simulink model "simulink_computer_auto_highlighted"  (R2022b)
settings: Solver=VariableStepAuto  StartTime=0.0  StopTime=inf  RelTol=1e-3
libraries: simulink_extras x21, dspswit3 x1, simulink x1, hdlsllib x1
(part 1 of 2)
settings Model: Creator=F1  LastModifiedBy=Namratha
settings SolverCC: AlgebraicLoopSolver=TrustRegion
settings OptimizationCC: BooleanDataType=off
settings DebuggingCC: UnconnectedInputMsg=warning  UnconnectedOutputMsg=warning  UnconnectedLineMsg=warning  SFMachineParentedDataDiag=warning
settings ModelReferenceCC: EnableRefExpFcnMdlSchedulingChecks=on

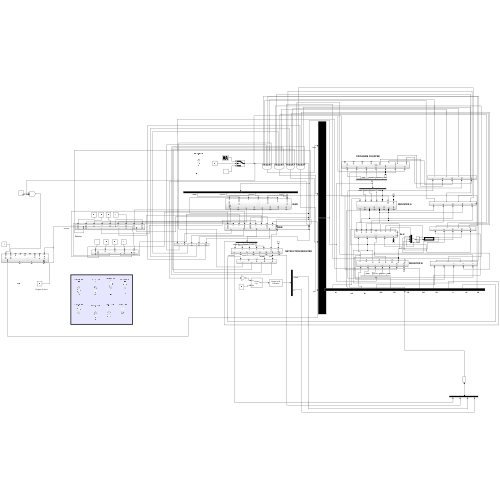
[thumbnail: Simulink's stored preview of the top-level diagram]
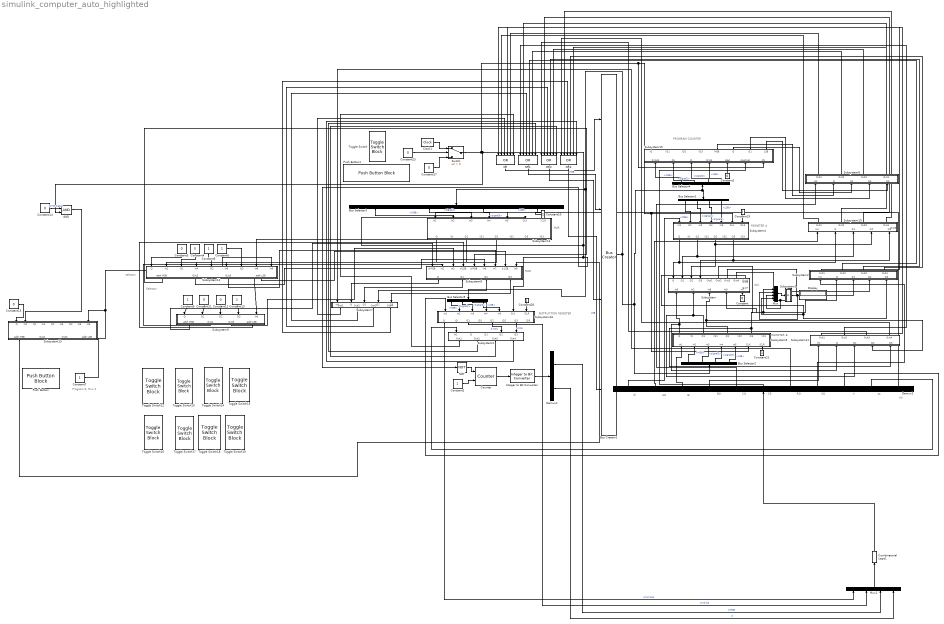
== system simulink_computer_auto_highlighted ==
  note: selector
  note: MI
  note: IO
  note: II
  note: SO
  note: RO
  note: CE
  note: CO
  note: BO
  note: BI
  note: AO
  note: AI
  note: MAR
  note: Program:0, Run:1
  note: ALU
  note: REGISTER B
  note: REGISTER A
  note: PROGRAM COUNTER
  note: RAM
  note: Selector
  note: INSTRUCTION REGISTER
  AND : Logic  IconShape=distinctive  AllPortsSameDT=off  OutDataTypeStr=boolean
  Bus Creator1 : BusCreator  Inputs=4
  Bus Selector{1..5} (5 alike) : BusSelector  OutputSignals=MSB,signal2,signal3,LSB
  Clock1 : simulink_extras/Flip Flops/Clock  period=2
  Combinatorial Logic1 : CombinatorialLogic  TruthTable=|
      | [0	0	0	0	1	0	0	0	0	0	1;
      | 0	0	0	0	0	1	1	0	1	0	0;
      | 0	0	0	0	0	0	0	0	0	1	1;
      | 1	0	0	0	0	0	1	0	0	0	0;
      | 0	0	0	0	1	0	0	0	0	0	1;
      | 0	0	0	0	0	1	1	0	1	0	0;
      | 0	0	1	0	0	0	0	0	0	1	0;
      | 0	0	0	0	0	0	0	0	0	0	0;
      | 0	0	0	0	1	0	0	0	0	0	1;
      | 0	0	0	0	0	1	1	0	1	0	0;
      | 0	0	1	0	0	0	0	1	0	0	0;
      | 0	0	0	0	0	0	0	0	0	0	0;
      | 0	0	0	0	0	0	0	0	0	0	0;
      | 0	0	0	0	0	0	0	0	0	0	0;
      | 0	0	0	0	0	0	0	0	0	0	0;
      | 0	0	0	0	0	0	0	0	0	0	0]
  Constant{,1,14..15,17,23} (6 alike) : Constant  Value=0
  Constant{2,10,19,21,28} (5 alike) : Constant
  Constant{3..4,11..12} (4 alike) : Constant  Value=0  OutDataTypeStr=boolean  LockScale=on
  Constant{5..7,9,13} (5 alike) : Constant  OutDataTypeStr=boolean  LockScale=on
  Counter : dspswit3/Counter  Direction=Up  CountEvent=Rising edge  CounterSize=User defined  MaxCount=3  InitialCount=0  Output=Count  HitValue=32  ResetInput=on  SamplesPerFrame=1  Ts=1  CntDtype=int16  HitDtype=Logical
  Demux1 : Demux  Outputs=2
  Demux2 : Demux  Outputs=11
  Display : Display
  Integer to Bit Converter : simulink/Logic and Bit Operations/Integer to Bit Converter  nbits=2  signedInputValues=Unsigned  bitOrder=MSB first  outDtype=boolean
      settings: LibrarySourceBlock=|
      | commutil2/Integer to Bit
      | Converter
  Mux : Mux
  Mux1 : Mux
  NOT : Logic  Operator=NOT  IconShape=distinctive  AllPortsSameDT=off  OutDataTypeStr=boolean
  OR{,1..3} (4 alike) : Logic  Operator=OR  Inputs=6  IconShape=distinctive  AllPortsSameDT=off  OutDataTypeStr=boolean
  Push Button : PushButtonBlock  OffValue=0.000000
  Push Button1 : PushButtonBlock  OffValue=0.000000
  Subsystem : Subsystem
      settings: PortSchema="{\"entries\":[{\"content\":{\"sides\":[{\"content\":{\"connectorIds\":[\"In1\",\"In2\",\"In3\",\"In4\",\"In5\"]},\"type\":\"ConnectorPlacement.EquallySpacedRectSide\",\"uuid\":\"d76b9681-1e35-4330-834d-a6fb8ece3ca6\"},{\"content\":{\"connectorIds\":[\"In6\",\"In7\",\"In8\",\"In9\",\"Out1\",\"Out2\",\"Out3\",\"Out4\",\"Out5\"],\"side\":\"RIGHT\"},\"type\":\"ConnectorPlacement.EquallySpacedRectSide\",\"uuid\":\"5f7e2d0d-b340-42cb-b0df-c47f3adaa3c8\"},{\"content\":{\"connectorIds\":[],\"side\":\"TOP\"},\"type\":\"ConnectorPlacement.EquallySpacedRectSide\",\"uuid\":\"9ba6019d-435d-4d43-af51-5a6472d9473c\"},{\"content\":{\"connectorIds\":[\"Out6\",\"Out7\"],\"side\":\"BOTTOM\"},\"type\":\"ConnectorPlacement.EquallySpacedRectSide\",\"uuid\":\"ff52050d-6b1c-4dc9-b693-b127a6983cae\"}]},\"type\":\"ConnectorPlacement.EquallySpacedConnector\",\"uuid\":\"63f40923-5384-474a-9ba8-b1a2be7f0fa2\"}],\"packageUris\":[\"http://schema.mathworks.com/mf0/Connector/R2020b\"],\"version\":\"1.0\"}"
  Subsystem1 : Subsystem
  Subsystem10 : Subsystem
      settings: PortSchema="{\"entries\":[{\"content\":{\"sides\":[{\"content\":{\"connectorIds\":[\"In1\",\"In2\",\"In3\",\"In4\",\"In5\"]},\"type\":\"ConnectorPlacement.EquallySpacedRectSide\",\"uuid\":\"be1d6c7a-a71e-4dd8-8c15-a91081576af0\"},{\"content\":{\"connectorIds\":[\"Out1\",\"Out2\",\"Out3\",\"Out4\"],\"side\":\"RIGHT\"},\"type\":\"ConnectorPlacement.EquallySpacedRectSide\",\"uuid\":\"047de8eb-1583-4af5-9052-d7fc7813080f\"},{\"content\":{\"connectorIds\":[],\"side\":\"TOP\"},\"type\":\"ConnectorPlacement.EquallySpacedRectSide\",\"uuid\":\"384f979b-6520-4a26-a075-1614f2aab292\"},{\"content\":{\"connectorIds\":[\"Out5\"],\"side\":\"BOTTOM\"},\"type\":\"ConnectorPlacement.EquallySpacedRectSide\",\"uuid\":\"fda4a962-651a-4873-b6d0-34c5738e96d2\"}]},\"type\":\"ConnectorPlacement.EquallySpacedConnector\",\"uuid\":\"d67f7e62-ac02-4d91-8456-d744cd866721\"}],\"packageUris\":[\"http://schema.mathworks.com/mf0/Connector/R2020b\"],\"version\":\"1.0\"}"
  Subsystem11 : Subsystem
  Subsystem12 : Subsystem
  Subsystem13 : Subsystem
  Subsystem14 : Subsystem
  Subsystem15 : Subsystem
  Subsystem16 : Subsystem
  Subsystem2 : Subsystem
  Subsystem3 : Subsystem
  Subsystem4 : Subsystem
  Subsystem5 : Subsystem
  Subsystem6 : Subsystem
  Subsystem7 : Subsystem
  Subsystem8 : Subsystem
  Subsystem9 : Subsystem
  Switch : Switch  Criteria=u2 > Threshold  SaturateOnIntegerOverflow=off  InputSameDT=off
  Toggle Switch{,12..19} (9 alike) : ToggleSwitchBlock
      settings: Values={{'Off', 'On'}, [0 1]}
  wires:
  Subsystem11/3(Out3) -> OR2/1
  Subsystem7/4(Out4) -> OR3/3
  Subsystem10/1(Out1) -> OR/2
  Subsystem11/4(Out4) -> OR3/1
  Subsystem4/3(Q1) -> Subsystem/7(Q1), Subsystem10/3(Q1)
  Bus Selector1/1 -> Subsystem4/2(In2)  "<MSB>"
  OR/1 -> Bus Creator1/1  "MSB"
  Subsystem7/1(Out1) -> OR/3
  Constant21/1 -> Subsystem5/7(!CLR)
  OR3/1 -> Bus Creator1/4  "LSB"
  Constant19/1 -> Subsystem4/7(!CLR)
  Bus Selector2/2 -> Subsystem5/3(In3)  "<signal2>"
  Bus Selector2/4 -> Subsystem5/5(In5)  "<LSB>"
  Bus Selector1/2 -> Subsystem4/3(In3)  "<signal2>"
  OR1/1 -> Bus Creator1/2
  Bus Selector1/3 -> Subsystem4/4(In4)  "<signal3>"
  Subsystem4/1(Q) -> Subsystem/6(Q), Subsystem10/2(Q)
  Subsystem7/2(Out2) -> OR1/3
  Subsystem7/3(Out3) -> OR2/3
  Subsystem10/4(Out4) -> OR3/2
  Subsystem4/7(Q3) -> Subsystem/9(Q3), Subsystem10/5(Q3)
  Subsystem5/7(Q3) -> Subsystem/4(In9), Subsystem11/5(Q3)
  Subsystem10/3(Out3) -> OR2/2
  Subsystem4/5(Q2) -> Subsystem/8(Q2), Subsystem10/4(Q2)
  Subsystem10/2(Out2) -> OR1/2
  Subsystem11/1(Out1) -> OR/1
  Subsystem5/5(Q2) -> Subsystem/3(In8), Subsystem11/4(Q2)
  Bus Selector2/1 -> Subsystem5/2(In2)  "<MSB>"
  Bus Selector1/4 -> Subsystem4/5(In5)  "<LSB>"
  Bus Selector2/3 -> Subsystem5/4(In4)  "<signal3>"
  Subsystem5/1(Q) -> Subsystem/1(In6), Subsystem11/2(Q)
  Subsystem5/3(Q1) -> Subsystem11/3(Q1), Subsystem/2(In2)
  OR2/1 -> Bus Creator1/3
  Subsystem11/2(Out2) -> OR1/1
  Constant/1 -> Subsystem/5(In7)
  Subsystem/2(Out2) -> Subsystem2/2(Q), Mux/1
  Subsystem/3(Out3) -> Mux/2, Subsystem2/3(Q1)
  Subsystem/4(Out4) -> Subsystem2/4(Q2), Mux/3
  Subsystem/5(Out5) -> Subsystem2/5(Q3), Mux/4
  Mux/1 -> Subsystem1/1(In1)
  Subsystem1/1(y) -> Display/1
  Demux2/8 -> Subsystem2/1(In1)
  Subsystem2/1(Out1) -> OR/4
  Subsystem2/2(Out2) -> OR1/4
  Subsystem2/3(Out3) -> OR2/4
  Subsystem2/4(Out4) -> OR3/4
  Subsystem6/4(Out4) -> OR3/5
  Subsystem6/3(Out3) -> OR2/5
  Subsystem6/2(Out2) -> OR1/5
  Subsystem6/1(Out1) -> OR/5
  Subsystem12/2(Out2) -> Subsystem8/6(In6)
  Subsystem12/4(addr LSB) -> Subsystem8/8(a LSB)
  Subsystem12/3(Out3) -> Subsystem8/7(In7)
  Subsystem12/1(addr MSB) -> Subsystem8/5(a MSB)
  Constant3/1 -> Subsystem12/1(Q)
  Constant4/1 -> Subsystem12/3(Q1)
  Constant5/1 -> Subsystem12/5(Q2)
  Constant6/1 -> Subsystem12/7(Q3)
  Bus Selector3/1 -> Subsystem14/2(In2)  "<MSB>"
  Bus Selector3/4 -> Subsystem14/5(In5)  "<LSB>"
  Bus Selector3/2 -> Subsystem14/3(In3)  "<signal2>"
  Bus Selector3/3 -> Subsystem14/4(In4)  "<signal3>"
  Subsystem14/1(Q) -> Subsystem12/2(In2)
  Subsystem14/3(Q1) -> Subsystem12/4(In4)
  Subsystem14/5(Q2) -> Subsystem12/6(In6)
  Subsystem14/7(Q3) -> Subsystem12/8(In8)
  Constant7/1 -> Subsystem13/9(In9), Subsystem9/5(In9), Subsystem12/9(In9)
  Constant10/1 -> Subsystem14/7(!CLR)
  Subsystem9/1(addr MSB) -> Subsystem8/1(d MSB)
  Subsystem9/2(Out2) -> Subsystem8/2(In2)
  Subsystem9/3(Out3) -> Subsystem8/3(In3)
  Subsystem9/4(addr LSB) -> Subsystem8/4(d LSB)
  Constant9/1 -> Subsystem9/1(Q)
  Constant11/1 -> Subsystem9/2(Q1)
  Constant12/1 -> Subsystem9/3(Q2)
  Constant13/1 -> Subsystem9/4(Q3)
  Constant15/1 -> Subsystem13/1(Q)
  Constant14/1 -> AND/1  "Write signal"
  AND/1 -> Subsystem13/2(In2)
  Subsystem13/1(addr MSB) -> Subsystem8/9(In9)
  Constant17/1 -> Switch/3
  Clock1/1 -> Switch/1
  Constant23/1 -> Switch/2
  Subsystem15/5(MSB) -> Subsystem6/2(Q)
  Subsystem15/6(Q) -> Subsystem6/3(Q1)
  Subsystem15/7(Q1) -> Subsystem6/4(Q2)
  Subsystem15/8(LSB) -> Subsystem6/5(Q3)
  Bus Selector4/1 -> Subsystem15/1(D msb)  "<MSB>"
  Bus Selector4/2 -> Subsystem15/2(D1)  "<signal2>"
  Bus Selector4/3 -> Subsystem15/3(D)  "<signal3>"
  Bus Selector4/4 -> Subsystem15/4(D lsb)  "<LSB>"
  Subsystem8/2(Q1) -> Subsystem7/3(Q1)
  Subsystem8/3(Q2) -> Subsystem7/4(Q2)
  Subsystem8/4(Q3) -> Subsystem7/5(Q3)
  Constant28/1 -> Subsystem16/7(!CLR)
  Bus Selector5/3 -> Subsystem16/4(In4)  "<signal3>"
  Bus Selector5/2 -> Subsystem16/3(In3)  "<signal2>"
  Bus Selector5/1 -> Subsystem16/2(In2)  "<MSB>"
  Bus Selector5/4 -> Subsystem16/5(In5)  "<LSB>"
  Subsystem16/5(Q2) -> Subsystem3/4(Q2)  "d msb"
  Subsystem16/7(Q3) -> Subsystem3/5(Q3)  "d lsb"
  Switch/1 -> Subsystem14/6(CLK), Subsystem16/6(CLK), NOT/1, AND/2, Subsystem4/6(CLK), Subsystem5/6(CLK), Subsystem15/7(clk)
  Bus Creator1/1 -> Bus Selector1/1, Bus Selector4/1, Bus Selector2/1, Bus Selector5/1, Bus Selector3/1
  Subsystem3/1(Out1) -> OR/6
  Subsystem3/2(Out2) -> OR1/6
  Subsystem3/3(Out3) -> OR2/6
  Subsystem3/4(Out4) -> OR3/6
  Counter/1 -> Integer to Bit Converter/1
  Integer to Bit Converter/1 -> Demux1/1
  Combinatorial Logic1/1 -> Demux2/1
  Mux1/1 -> Combinatorial Logic1/1
  NOT/1 -> Counter/1
  Constant2/1 -> Counter/2
  Demux1/1 -> Mux1/3  "d MSB"
  Demux1/2 -> Mux1/4  "d"
  Subsystem16/1(Q) -> Mux1/1  "cmd msb"
  Subsystem16/3(Q1) -> Mux1/2  "cmd lsb"
  Demux2/3 -> Subsystem5/1(In1)
  Demux2/1 -> Subsystem4/1(In1)
  Demux2/4 -> Subsystem11/1(In1)
  Demux2/2 -> Subsystem10/1(In1)
  Demux2/6 -> Subsystem15/6(count en)
  Demux2/5 -> Subsystem6/1(In1)
  Demux2/7 -> Subsystem7/1(In1)
  Subsystem8/1(Q) -> Subsystem7/2(Q)
  Demux2/9 -> Subsystem16/1(In1)
  Demux2/11 -> Subsystem14/1(In1)
  Demux2/10 -> Subsystem3/1(In1)
  Constant1/1 -> Subsystem15/5(load)

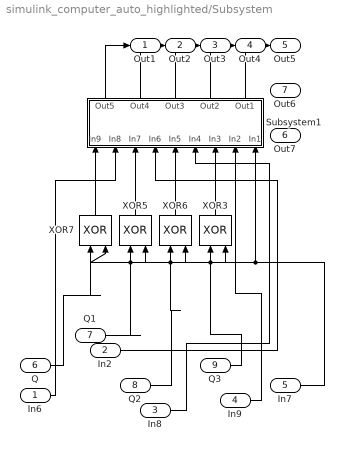
== system simulink_computer_auto_highlighted/Subsystem ==
  In6 : Inport
  In2 : Inport  Port=2
  In8 : Inport  Port=3
  In9 : Inport  Port=4
  In7 : Inport  Port=5
  Q : Inport  Port=6
  Q1 : Inport  Port=7
  Q2 : Inport  Port=8
  Q3 : Inport  Port=9
  Subsystem1 : Subsystem
  XOR{3,5..7} (4 alike) : Logic  Operator=XOR  IconShape=distinctive  AllPortsSameDT=off  OutDataTypeStr=boolean
  Out1 : Outport
  Out2 : Outport  Port=2
  Out3 : Outport  Port=3
  Out4 : Outport  Port=4
  Out5 : Outport  Port=5
  Out7 : Outport  Port=6
  Out6 : Outport  Port=7
  wires:
  XOR6/1 -> Subsystem1/5(In5)
  XOR5/1 -> Subsystem1/7(In7)
  XOR3/1 -> Subsystem1/3(In3)
  Subsystem1/1(Out1) -> Out5/1
  In7/1 -> XOR7/1, XOR5/1, XOR6/1, XOR3/1, Subsystem1/1(In1)
  Subsystem1/2(Out2) -> Out4/1
  Subsystem1/4(Out4) -> Out2/1
  Subsystem1/3(Out3) -> Out3/1
  In2/1 -> Subsystem1/6(In6)
  XOR7/1 -> Subsystem1/9(In9)
  Subsystem1/5(Out5) -> Out1/1
  Q3/1 -> XOR3/2
  Q1/1 -> XOR5/2
  Q/1 -> XOR7/2
  In6/1 -> Subsystem1/8(In8)
  In9/1 -> Subsystem1/2(In2)
  Q2/1 -> XOR6/2
  In8/1 -> Subsystem1/4(In4)

== system simulink_computer_auto_highlighted/Subsystem1 ==
  In1 : Inport
  Demux : Demux
  MATLAB Function : MATLAB Function  TreatAsAtomicUnit=on
  y : Outport
  wires:
  Demux/3 -> MATLAB Function/3(b1)
  Demux/1 -> MATLAB Function/1(b3)
  Demux/2 -> MATLAB Function/2(b2)
  Demux/4 -> MATLAB Function/4(b0)
  MATLAB Function/1(y) -> y/1
  In1/1 -> Demux/1

== system simulink_computer_auto_highlighted/Subsystem10 ==
  In1 : Inport
  Q : Inport  Port=2
  Q1 : Inport  Port=3
  Q2 : Inport  Port=4
  Q3 : Inport  Port=5
  AND{,1..3} (4 alike) : Logic  IconShape=distinctive  AllPortsSameDT=off  OutDataTypeStr=boolean
  Out1 : Outport
  Out2 : Outport  Port=2
  Out3 : Outport  Port=3
  Out4 : Outport  Port=4
  Out5 : Outport  Port=5
  wires:
  In1/1 -> AND3/1, AND2/1, AND1/1, AND/1
  AND1/1 -> Out2/1
  AND3/1 -> Out4/1
  AND/1 -> Out1/1
  Q3/1 -> AND3/2
  Q2/1 -> AND2/2
  Q/1 -> AND/2
  AND2/1 -> Out3/1
  Q1/1 -> AND1/2

== system simulink_computer_auto_highlighted/Subsystem11 ==
  In1 : Inport
  Q : Inport  Port=2
  Q1 : Inport  Port=3
  Q2 : Inport  Port=4
  Q3 : Inport  Port=5
  AND{,1..3} (4 alike) : Logic  IconShape=distinctive  AllPortsSameDT=off  OutDataTypeStr=boolean
  Out1 : Outport
  Out2 : Outport  Port=2
  Out3 : Outport  Port=3
  Out4 : Outport  Port=4
  wires:
  In1/1 -> AND3/1, AND2/1, AND1/1, AND/1
  AND1/1 -> Out2/1
  AND3/1 -> Out4/1
  AND/1 -> Out1/1
  Q3/1 -> AND3/2
  Q2/1 -> AND2/2
  Q/1 -> AND/2
  AND2/1 -> Out3/1
  Q1/1 -> AND1/2

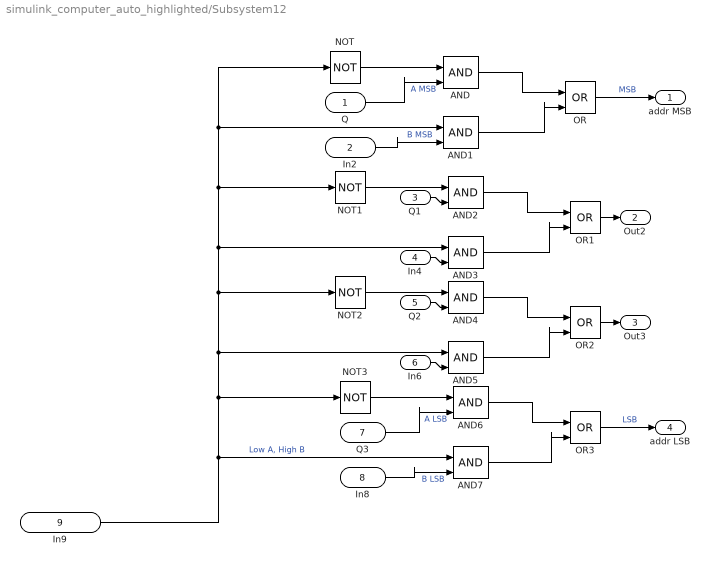
== system simulink_computer_auto_highlighted/Subsystem12 ==
  Q : Inport
  In2 : Inport  Port=2
  Q1 : Inport  Port=3
  In4 : Inport  Port=4
  Q2 : Inport  Port=5
  In6 : Inport  Port=6
  Q3 : Inport  Port=7
  In8 : Inport  Port=8
  In9 : Inport  Port=9
  AND{,1..7} (8 alike) : Logic  IconShape=distinctive  AllPortsSameDT=off  OutDataTypeStr=boolean
  NOT{,1..3} (4 alike) : Logic  Operator=NOT  IconShape=distinctive  AllPortsSameDT=off  OutDataTypeStr=boolean
  OR{,1..3} (4 alike) : Logic  Operator=OR  IconShape=distinctive  AllPortsSameDT=off  OutDataTypeStr=boolean
  addr MSB : Outport
  Out2 : Outport  Port=2
  Out3 : Outport  Port=3
  addr LSB : Outport  Port=4
  wires:
  In9/1 -> AND7/1, NOT3/1, AND5/1, NOT2/1, NOT1/1, AND1/1, NOT/1, AND3/1  "Low A, High B"
  AND5/1 -> OR2/2
  NOT/1 -> AND/1
  NOT1/1 -> AND2/1
  AND/1 -> OR/1
  AND2/1 -> OR1/1
  In4/1 -> AND3/2
  NOT2/1 -> AND4/1
  AND3/1 -> OR1/2
  AND4/1 -> OR2/1
  OR1/1 -> Out2/1
  Q2/1 -> AND4/2
  AND7/1 -> OR3/2
  AND1/1 -> OR/2
  OR/1 -> addr MSB/1  "MSB"
  AND6/1 -> OR3/1
  Q1/1 -> AND2/2
  OR2/1 -> Out3/1
  NOT3/1 -> AND6/1
  In2/1 -> AND1/2  "B MSB"
  In6/1 -> AND5/2
  Q/1 -> AND/2  "A MSB"
  In8/1 -> AND7/2  "B LSB"
  Q3/1 -> AND6/2  "A LSB"
  OR3/1 -> addr LSB/1  "LSB"

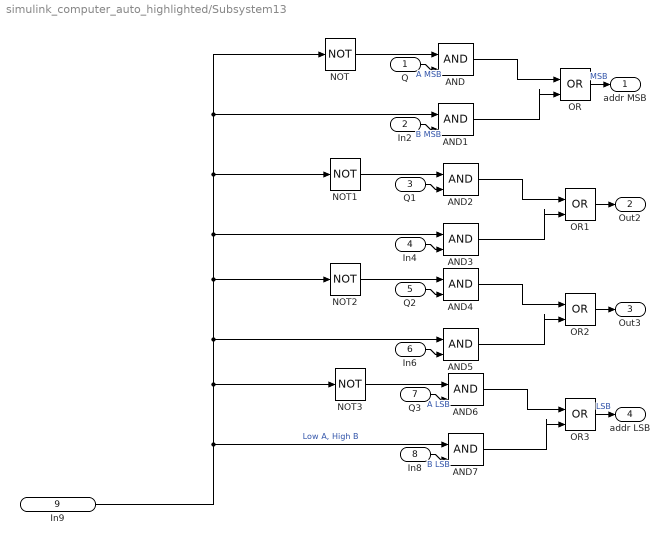
== system simulink_computer_auto_highlighted/Subsystem13 ==
  Q : Inport
  In2 : Inport  Port=2
  Q1 : Inport  Port=3
  In4 : Inport  Port=4
  Q2 : Inport  Port=5
  In6 : Inport  Port=6
  Q3 : Inport  Port=7
  In8 : Inport  Port=8
  In9 : Inport  Port=9
  AND{,1..7} (8 alike) : Logic  IconShape=distinctive  AllPortsSameDT=off  OutDataTypeStr=boolean
  NOT{,1..3} (4 alike) : Logic  Operator=NOT  IconShape=distinctive  AllPortsSameDT=off  OutDataTypeStr=boolean
  OR{,1..3} (4 alike) : Logic  Operator=OR  IconShape=distinctive  AllPortsSameDT=off  OutDataTypeStr=boolean
  addr MSB : Outport
  Out2 : Outport  Port=2
  Out3 : Outport  Port=3
  addr LSB : Outport  Port=4
  wires:
  In9/1 -> AND7/1, NOT3/1, AND5/1, NOT2/1, NOT1/1, AND1/1, NOT/1, AND3/1  "Low A, High B"
  AND5/1 -> OR2/2
  NOT/1 -> AND/1
  NOT1/1 -> AND2/1
  AND/1 -> OR/1
  AND2/1 -> OR1/1
  In4/1 -> AND3/2
  NOT2/1 -> AND4/1
  AND3/1 -> OR1/2
  AND4/1 -> OR2/1
  OR1/1 -> Out2/1
  Q2/1 -> AND4/2
  AND7/1 -> OR3/2
  AND1/1 -> OR/2
  OR/1 -> addr MSB/1  "MSB"
  AND6/1 -> OR3/1
  Q1/1 -> AND2/2
  OR2/1 -> Out3/1
  NOT3/1 -> AND6/1
  In2/1 -> AND1/2  "B MSB"
  In6/1 -> AND5/2
  Q/1 -> AND/2  "A MSB"
  In8/1 -> AND7/2  "B LSB"
  Q3/1 -> AND6/2  "A LSB"
  OR3/1 -> addr LSB/1  "LSB"

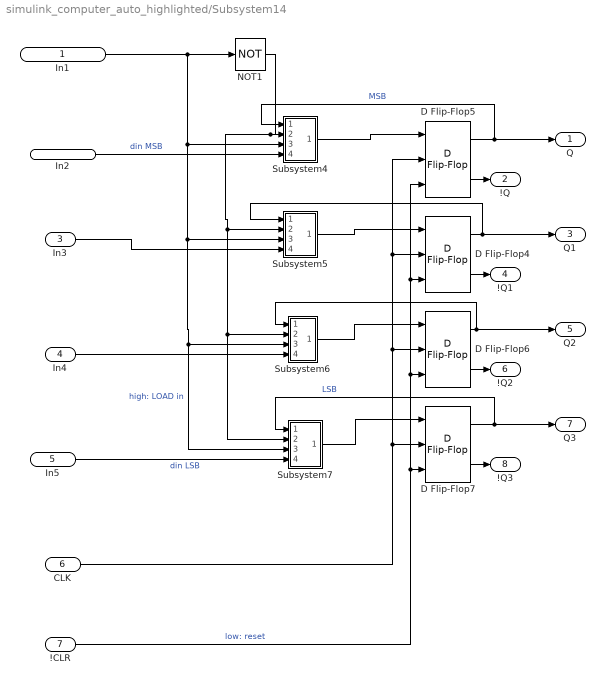
== system simulink_computer_auto_highlighted/Subsystem14 ==
  In1 : Inport
  In2 : Inport  Port=2
  In3 : Inport  Port=3
  In4 : Inport  Port=4
  In5 : Inport  Port=5
  CLK : Inport  Port=6
  !CLR : Inport  Port=7
  D Flip-Flop{4..7} (4 alike) : simulink_extras/Flip Flops/D Flip-Flop
  NOT1 : Logic  Operator=NOT  IconShape=distinctive  AllPortsSameDT=off  OutDataTypeStr=boolean
  Subsystem4 : Subsystem
  Subsystem5 : Subsystem
  Subsystem6 : Subsystem
  Subsystem7 : Subsystem
  Q : Outport
  !Q : Outport  Port=2
  Q1 : Outport  Port=3
  !Q1 : Outport  Port=4
  Q2 : Outport  Port=5
  !Q2 : Outport  Port=6
  Q3 : Outport  Port=7
  !Q3 : Outport  Port=8
  wires:
  In5/1 -> Subsystem7/4(In4)  "din LSB"
  D Flip-Flop5/1 -> Q/1, Subsystem4/1(In1)  "MSB"
  NOT1/1 -> Subsystem7/2(In2), Subsystem6/2(In2), Subsystem5/2(In1), Subsystem4/2(In2)
  Subsystem4/1(Out1) -> D Flip-Flop5/1
  Subsystem7/1(Out1) -> D Flip-Flop7/1
  In3/1 -> Subsystem5/4(In4)
  D Flip-Flop4/2 -> !Q1/1
  D Flip-Flop4/1 -> Q1/1, Subsystem5/1(In2)
  D Flip-Flop7/2 -> !Q3/1
  D Flip-Flop7/1 -> Q3/1, Subsystem7/1(In1)  "LSB"
  D Flip-Flop5/2 -> !Q/1
  Subsystem5/1(Out1) -> D Flip-Flop4/1
  D Flip-Flop6/2 -> !Q2/1
  Subsystem6/1(Out1) -> D Flip-Flop6/1
  D Flip-Flop6/1 -> Q2/1, Subsystem6/1(In1)
  In1/1 -> Subsystem7/3(In3), Subsystem6/3(In3), Subsystem5/3(In3), Subsystem4/3(In3), NOT1/1  "high: LOAD in"
  !CLR/1 -> D Flip-Flop5/3, D Flip-Flop4/3, D Flip-Flop6/3, D Flip-Flop7/3  "low: reset"
  CLK/1 -> D Flip-Flop5/2, D Flip-Flop4/2, D Flip-Flop6/2, D Flip-Flop7/2
  In2/1 -> Subsystem4/4(In4)  "din MSB"
  In4/1 -> Subsystem6/4(In4)

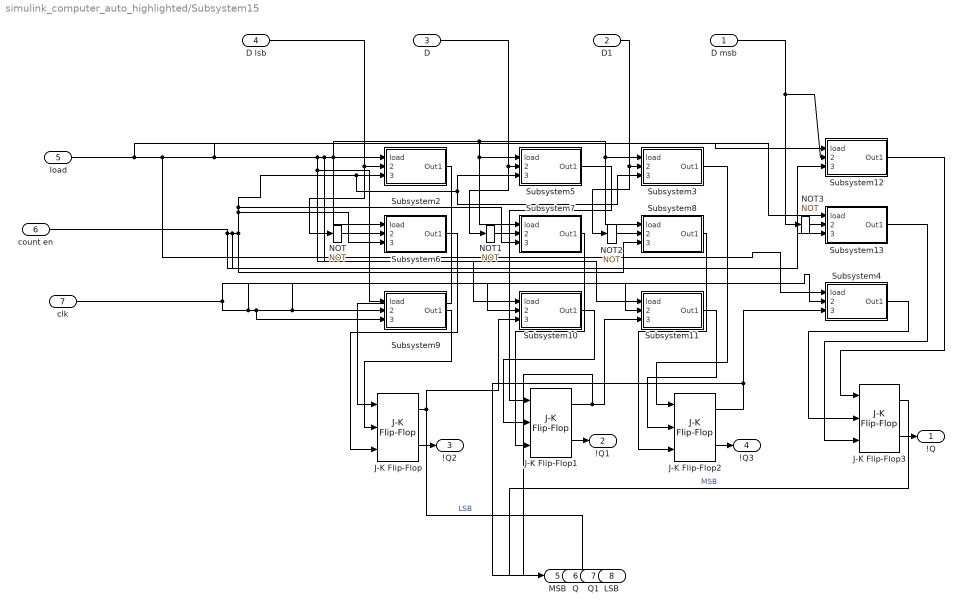
== system simulink_computer_auto_highlighted/Subsystem15 ==
  D msb : Inport
  D1 : Inport  Port=2
  D : Inport  Port=3
  D lsb : Inport  Port=4
  load : Inport  Port=5
  count en : Inport  Port=6
  clk : Inport  Port=7
  J-K Flip-Flop{,1..3} (4 alike) : simulink_extras/Flip Flops/J-K Flip-Flop  initial_condition=0
  NOT{,1..3} (4 alike) : Logic  Operator=NOT  IconShape=distinctive  AllPortsSameDT=off  OutDataTypeStr=boolean
  Subsystem10 : Subsystem
  Subsystem11 : Subsystem
  Subsystem12 : Subsystem
  Subsystem13 : Subsystem
  Subsystem2 : Subsystem
  Subsystem3 : Subsystem
  Subsystem4 : Subsystem
  Subsystem5 : Subsystem
  Subsystem6 : Subsystem
  Subsystem7 : Subsystem
  Subsystem8 : Subsystem
  Subsystem9 : Subsystem
  !Q : Outport
  !Q1 : Outport  Port=2
  !Q2 : Outport  Port=3
  !Q3 : Outport  Port=4
  MSB : Outport  Port=5
  Q : Outport  Port=6
  Q1 : Outport  Port=7
  LSB : Outport  Port=8
  wires:
  count en/1 -> Subsystem12/3(select low), Subsystem13/3(select low), Subsystem5/3(select low), Subsystem3/3(select low), Subsystem2/3(select low), Subsystem7/3(select low), Subsystem6/3(select low), Subsystem8/3(select low)
  clk/1 -> Subsystem11/2(select high), Subsystem9/3(select low), Subsystem4/2(select high), Subsystem9/2(select high), Subsystem10/2(select high)
  Subsystem4/1(Out1) -> J-K Flip-Flop3/2
  Subsystem9/1(Out1) -> J-K Flip-Flop/2
  NOT2/1 -> Subsystem8/2(select high)
  Subsystem13/1(Out1) -> J-K Flip-Flop3/3
  load/1 -> Subsystem13/1(load), Subsystem4/1(load), Subsystem12/1(load), Subsystem10/1(load), Subsystem9/1(load), Subsystem11/1(load), Subsystem7/1(load), Subsystem5/1(load), Subsystem8/1(load), Subsystem3/1(load), Subsystem2/1(load), Subsystem6/1(load)
  J-K Flip-Flop3/2 -> !Q/1
  J-K Flip-Flop3/1 -> MSB/1  "MSB"
  Subsystem2/1(Out1) -> J-K Flip-Flop/1
  Subsystem12/1(Out1) -> J-K Flip-Flop3/1
  NOT/1 -> Subsystem6/2(select high)
  D/1 -> NOT1/1, Subsystem5/2(select high)
  Subsystem3/1(Out1) -> J-K Flip-Flop2/1
  NOT1/1 -> Subsystem7/2(select high)
  D msb/1 -> NOT3/1, Subsystem12/2(select high)
  Subsystem6/1(Out1) -> J-K Flip-Flop/3
  D lsb/1 -> NOT/1, Subsystem2/2(select high)
  Subsystem8/1(Out1) -> J-K Flip-Flop2/3
  NOT3/1 -> Subsystem13/2(select high)
  Subsystem10/1(Out1) -> J-K Flip-Flop1/2
  Subsystem5/1(Out1) -> J-K Flip-Flop1/1
  J-K Flip-Flop/1 -> LSB/1, Subsystem10/3(select low)  "LSB"
  D1/1 -> NOT2/1, Subsystem3/2(select high)
  J-K Flip-Flop1/2 -> !Q1/1
  Subsystem7/1(Out1) -> J-K Flip-Flop1/3
  J-K Flip-Flop1/1 -> Q1/1, Subsystem11/3(select low)
  J-K Flip-Flop2/2 -> !Q3/1
  J-K Flip-Flop2/1 -> Q/1, Subsystem4/3(select low)
  Subsystem11/1(Out1) -> J-K Flip-Flop2/2
  J-K Flip-Flop/2 -> !Q2/1

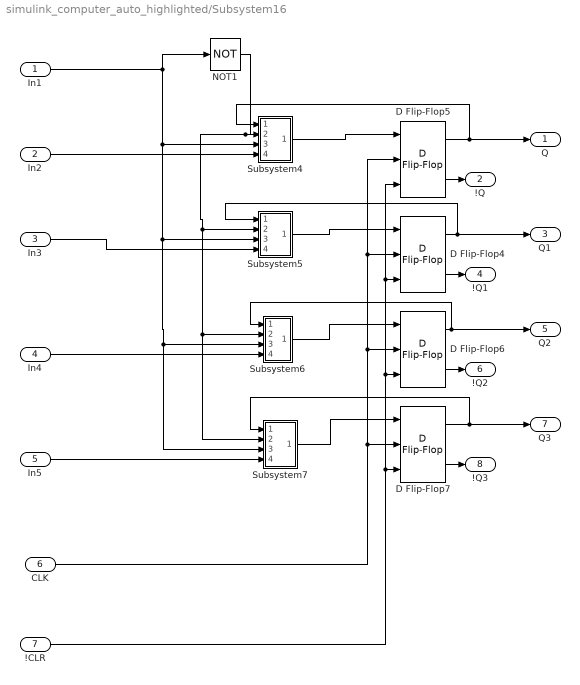
== system simulink_computer_auto_highlighted/Subsystem16 ==
  In1 : Inport
  In2 : Inport  Port=2
  In3 : Inport  Port=3
  In4 : Inport  Port=4
  In5 : Inport  Port=5
  CLK : Inport  Port=6
  !CLR : Inport  Port=7
  D Flip-Flop{4..7} (4 alike) : simulink_extras/Flip Flops/D Flip-Flop
  NOT1 : Logic  Operator=NOT  IconShape=distinctive  AllPortsSameDT=off  OutDataTypeStr=boolean
  Subsystem4 : Subsystem
  Subsystem5 : Subsystem
  Subsystem6 : Subsystem
  Subsystem7 : Subsystem
  Q : Outport
  !Q : Outport  Port=2
  Q1 : Outport  Port=3
  !Q1 : Outport  Port=4
  Q2 : Outport  Port=5
  !Q2 : Outport  Port=6
  Q3 : Outport  Port=7
  !Q3 : Outport  Port=8
  wires:
  In5/1 -> Subsystem7/4(In4)
  D Flip-Flop5/1 -> Q/1, Subsystem4/1(In1)
  NOT1/1 -> Subsystem7/2(In2), Subsystem6/2(In2), Subsystem5/2(In1), Subsystem4/2(In2)
  Subsystem4/1(Out1) -> D Flip-Flop5/1
  Subsystem7/1(Out1) -> D Flip-Flop7/1
  In3/1 -> Subsystem5/4(In4)
  D Flip-Flop4/2 -> !Q1/1
  D Flip-Flop4/1 -> Q1/1, Subsystem5/1(In2)
  D Flip-Flop7/2 -> !Q3/1
  D Flip-Flop7/1 -> Q3/1, Subsystem7/1(In1)
  D Flip-Flop5/2 -> !Q/1
  Subsystem5/1(Out1) -> D Flip-Flop4/1
  D Flip-Flop6/2 -> !Q2/1
  Subsystem6/1(Out1) -> D Flip-Flop6/1
  D Flip-Flop6/1 -> Q2/1, Subsystem6/1(In1)
  In1/1 -> NOT1/1, Subsystem7/3(In3), Subsystem6/3(In3), Subsystem5/3(In3), Subsystem4/3(In3)
  !CLR/1 -> D Flip-Flop5/3, D Flip-Flop4/3, D Flip-Flop6/3, D Flip-Flop7/3
  CLK/1 -> D Flip-Flop5/2, D Flip-Flop4/2, D Flip-Flop6/2, D Flip-Flop7/2
  In2/1 -> Subsystem4/4(In4)
  In4/1 -> Subsystem6/4(In4)

== system simulink_computer_auto_highlighted/Subsystem2 ==
  In1 : Inport
  Q : Inport  Port=2
  Q1 : Inport  Port=3
  Q2 : Inport  Port=4
  Q3 : Inport  Port=5
  AND{,1..3} (4 alike) : Logic  IconShape=distinctive  AllPortsSameDT=off  OutDataTypeStr=boolean
  Out1 : Outport
  Out2 : Outport  Port=2
  Out3 : Outport  Port=3
  Out4 : Outport  Port=4
  wires:
  In1/1 -> AND3/1, AND2/1, AND1/1, AND/1
  AND1/1 -> Out2/1
  AND3/1 -> Out4/1
  AND/1 -> Out1/1
  Q3/1 -> AND3/2
  Q2/1 -> AND2/2
  Q/1 -> AND/2
  AND2/1 -> Out3/1
  Q1/1 -> AND1/2

== system simulink_computer_auto_highlighted/Subsystem3 ==
  In1 : Inport
  Q : Inport  Port=2
  Q1 : Inport  Port=3
  Q2 : Inport  Port=4
  Q3 : Inport  Port=5
  AND{,1..3} (4 alike) : Logic  IconShape=distinctive  AllPortsSameDT=off  OutDataTypeStr=boolean
  Out1 : Outport
  Out2 : Outport  Port=2
  Out3 : Outport  Port=3
  Out4 : Outport  Port=4
  wires:
  In1/1 -> AND3/1, AND2/1, AND1/1, AND/1
  AND1/1 -> Out2/1
  AND3/1 -> Out4/1
  AND/1 -> Out1/1
  Q3/1 -> AND3/2
  Q2/1 -> AND2/2
  Q/1 -> AND/2
  AND2/1 -> Out3/1
  Q1/1 -> AND1/2

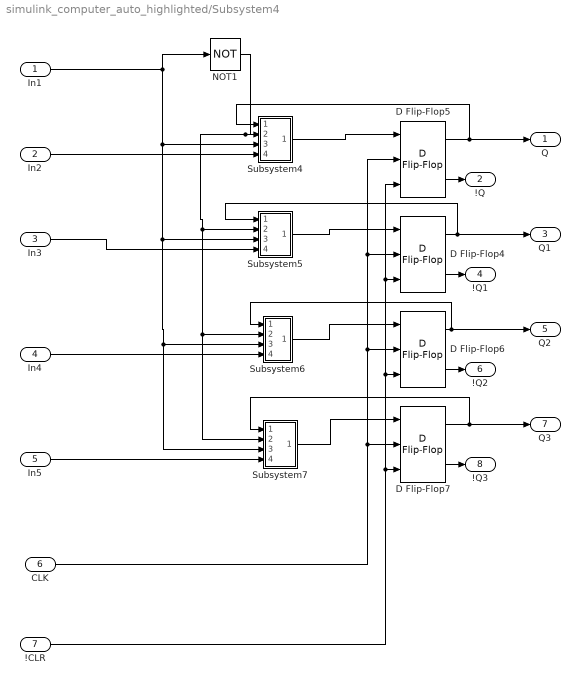
== system simulink_computer_auto_highlighted/Subsystem4 ==
  In1 : Inport
  In2 : Inport  Port=2
  In3 : Inport  Port=3
  In4 : Inport  Port=4
  In5 : Inport  Port=5
  CLK : Inport  Port=6
  !CLR : Inport  Port=7
  D Flip-Flop{4..7} (4 alike) : simulink_extras/Flip Flops/D Flip-Flop
  NOT1 : Logic  Operator=NOT  IconShape=distinctive  AllPortsSameDT=off  OutDataTypeStr=boolean
  Subsystem4 : Subsystem
  Subsystem5 : Subsystem
  Subsystem6 : Subsystem
  Subsystem7 : Subsystem
  Q : Outport
  !Q : Outport  Port=2
  Q1 : Outport  Port=3
  !Q1 : Outport  Port=4
  Q2 : Outport  Port=5
  !Q2 : Outport  Port=6
  Q3 : Outport  Port=7
  !Q3 : Outport  Port=8
  wires:
  In5/1 -> Subsystem7/4(In4)
  D Flip-Flop5/1 -> Q/1, Subsystem4/1(In1)
  NOT1/1 -> Subsystem7/2(In2), Subsystem6/2(In2), Subsystem5/2(In1), Subsystem4/2(In2)
  Subsystem4/1(Out1) -> D Flip-Flop5/1
  Subsystem7/1(Out1) -> D Flip-Flop7/1
  In3/1 -> Subsystem5/4(In4)
  D Flip-Flop4/2 -> !Q1/1
  D Flip-Flop4/1 -> Q1/1, Subsystem5/1(In2)
  D Flip-Flop7/2 -> !Q3/1
  D Flip-Flop7/1 -> Q3/1, Subsystem7/1(In1)
  D Flip-Flop5/2 -> !Q/1
  Subsystem5/1(Out1) -> D Flip-Flop4/1
  D Flip-Flop6/2 -> !Q2/1
  Subsystem6/1(Out1) -> D Flip-Flop6/1
  D Flip-Flop6/1 -> Q2/1, Subsystem6/1(In1)
  In1/1 -> NOT1/1, Subsystem7/3(In3), Subsystem6/3(In3), Subsystem5/3(In3), Subsystem4/3(In3)
  !CLR/1 -> D Flip-Flop5/3, D Flip-Flop4/3, D Flip-Flop6/3, D Flip-Flop7/3
  CLK/1 -> D Flip-Flop5/2, D Flip-Flop4/2, D Flip-Flop6/2, D Flip-Flop7/2
  In2/1 -> Subsystem4/4(In4)
  In4/1 -> Subsystem6/4(In4)

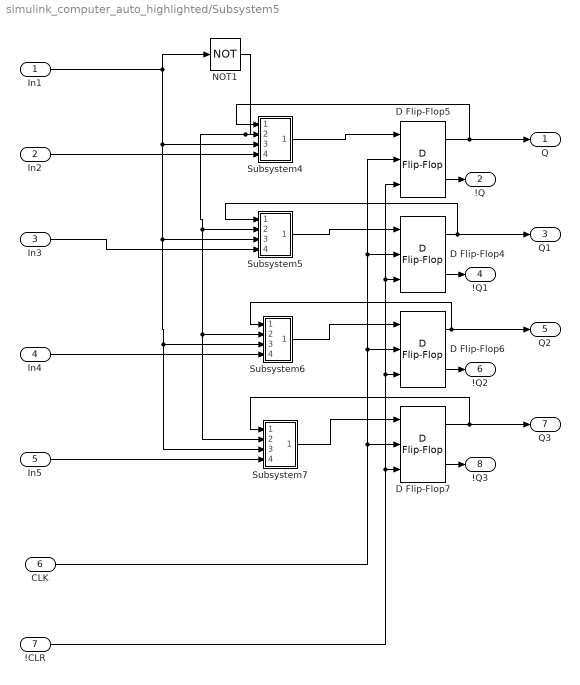
== system simulink_computer_auto_highlighted/Subsystem5 ==
  In1 : Inport
  In2 : Inport  Port=2
  In3 : Inport  Port=3
  In4 : Inport  Port=4
  In5 : Inport  Port=5
  CLK : Inport  Port=6
  !CLR : Inport  Port=7
  D Flip-Flop{4..7} (4 alike) : simulink_extras/Flip Flops/D Flip-Flop
  NOT1 : Logic  Operator=NOT  IconShape=distinctive  AllPortsSameDT=off  OutDataTypeStr=boolean
  Subsystem4 : Subsystem
  Subsystem5 : Subsystem
  Subsystem6 : Subsystem
  Subsystem7 : Subsystem
  Q : Outport
  !Q : Outport  Port=2
  Q1 : Outport  Port=3
  !Q1 : Outport  Port=4
  Q2 : Outport  Port=5
  !Q2 : Outport  Port=6
  Q3 : Outport  Port=7
  !Q3 : Outport  Port=8
  wires:
  In5/1 -> Subsystem7/4(In4)
  D Flip-Flop5/1 -> Q/1, Subsystem4/1(In1)
  NOT1/1 -> Subsystem7/2(In2), Subsystem6/2(In2), Subsystem5/2(In1), Subsystem4/2(In2)
  Subsystem4/1(Out1) -> D Flip-Flop5/1
  Subsystem7/1(Out1) -> D Flip-Flop7/1
  In3/1 -> Subsystem5/4(In4)
  D Flip-Flop4/2 -> !Q1/1
  D Flip-Flop4/1 -> Q1/1, Subsystem5/1(In2)
  D Flip-Flop7/2 -> !Q3/1
  D Flip-Flop7/1 -> Q3/1, Subsystem7/1(In1)
  D Flip-Flop5/2 -> !Q/1
  Subsystem5/1(Out1) -> D Flip-Flop4/1
  D Flip-Flop6/2 -> !Q2/1
  Subsystem6/1(Out1) -> D Flip-Flop6/1
  D Flip-Flop6/1 -> Q2/1, Subsystem6/1(In1)
  In1/1 -> NOT1/1, Subsystem7/3(In3), Subsystem6/3(In3), Subsystem5/3(In3), Subsystem4/3(In3)
  !CLR/1 -> D Flip-Flop5/3, D Flip-Flop4/3, D Flip-Flop6/3, D Flip-Flop7/3
  CLK/1 -> D Flip-Flop5/2, D Flip-Flop4/2, D Flip-Flop6/2, D Flip-Flop7/2
  In2/1 -> Subsystem4/4(In4)
  In4/1 -> Subsystem6/4(In4)

== system simulink_computer_auto_highlighted/Subsystem6 ==
  In1 : Inport
  Q : Inport  Port=2
  Q1 : Inport  Port=3
  Q2 : Inport  Port=4
  Q3 : Inport  Port=5
  AND{,1..3} (4 alike) : Logic  IconShape=distinctive  AllPortsSameDT=off  OutDataTypeStr=boolean
  Out1 : Outport
  Out2 : Outport  Port=2
  Out3 : Outport  Port=3
  Out4 : Outport  Port=4
  wires:
  In1/1 -> AND3/1, AND2/1, AND1/1, AND/1
  AND1/1 -> Out2/1
  AND3/1 -> Out4/1
  AND/1 -> Out1/1
  Q3/1 -> AND3/2
  Q2/1 -> AND2/2
  Q/1 -> AND/2
  AND2/1 -> Out3/1
  Q1/1 -> AND1/2

== system simulink_computer_auto_highlighted/Subsystem7 ==
  In1 : Inport
  Q : Inport  Port=2
  Q1 : Inport  Port=3
  Q2 : Inport  Port=4
  Q3 : Inport  Port=5
  AND{,1..3} (4 alike) : Logic  IconShape=distinctive  AllPortsSameDT=off  OutDataTypeStr=boolean
  Out1 : Outport
  Out2 : Outport  Port=2
  Out3 : Outport  Port=3
  Out4 : Outport  Port=4
  wires:
  In1/1 -> AND3/1, AND2/1, AND1/1, AND/1
  AND1/1 -> Out2/1
  AND3/1 -> Out4/1
  AND/1 -> Out1/1
  Q3/1 -> AND3/2
  Q2/1 -> AND2/2
  Q/1 -> AND/2
  AND2/1 -> Out3/1
  Q1/1 -> AND1/2

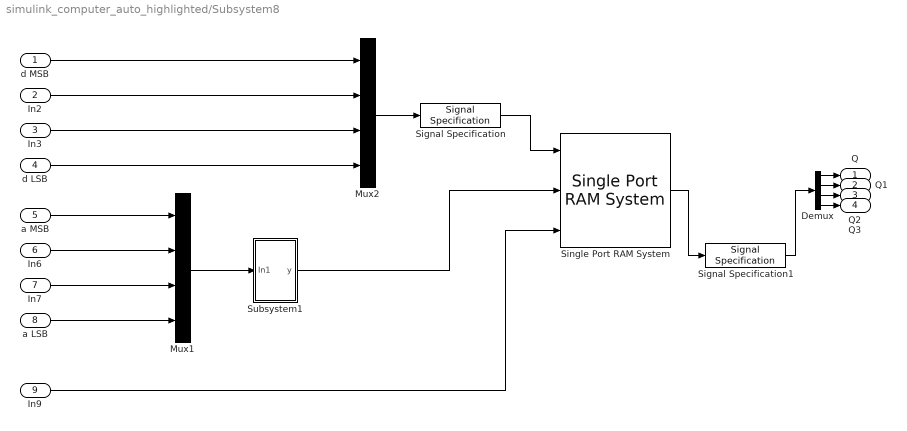
== system simulink_computer_auto_highlighted/Subsystem8 ==
  d MSB : Inport
  In2 : Inport  Port=2
  In3 : Inport  Port=3
  d LSB : Inport  Port=4
  a MSB : Inport  Port=5
  In6 : Inport  Port=6
  In7 : Inport  Port=7
  a LSB : Inport  Port=8
  In9 : Inport  Port=9
  Demux : Demux
  Mux1 : Mux
  Mux2 : Mux
  Signal Specification : SignalSpecification  Dimensions=[4 1]
  Signal Specification1 : SignalSpecification  Dimensions=[4 1]
  Single Port RAM System : hdlsllib/HDL RAMs/Single Port RAM System  RAMType=Single port  WriteOutputValue=New data  RAMInitialValue=0  SimulateUsing=Code generation
  Subsystem1 : Subsystem
  Q : Outport
  Q1 : Outport  Port=2
  Q2 : Outport  Port=3
  Q3 : Outport  Port=4
  wires:
  a LSB/1 -> Mux1/4
  In7/1 -> Mux1/3
  In2/1 -> Mux2/2
  a MSB/1 -> Mux1/1
  Subsystem1/1(y) -> Single Port RAM System/2
  d LSB/1 -> Mux2/4
  d MSB/1 -> Mux2/1
  In9/1 -> Single Port RAM System/3
  Mux1/1 -> Subsystem1/1(In1)
  Demux/1 -> Q/1
  In3/1 -> Mux2/3
  In6/1 -> Mux1/2
  Demux/2 -> Q1/1
  Demux/3 -> Q2/1
  Demux/4 -> Q3/1
  Single Port RAM System/1 -> Signal Specification1/1
  Signal Specification/1 -> Single Port RAM System/1
  Mux2/1 -> Signal Specification/1
  Signal Specification1/1 -> Demux/1

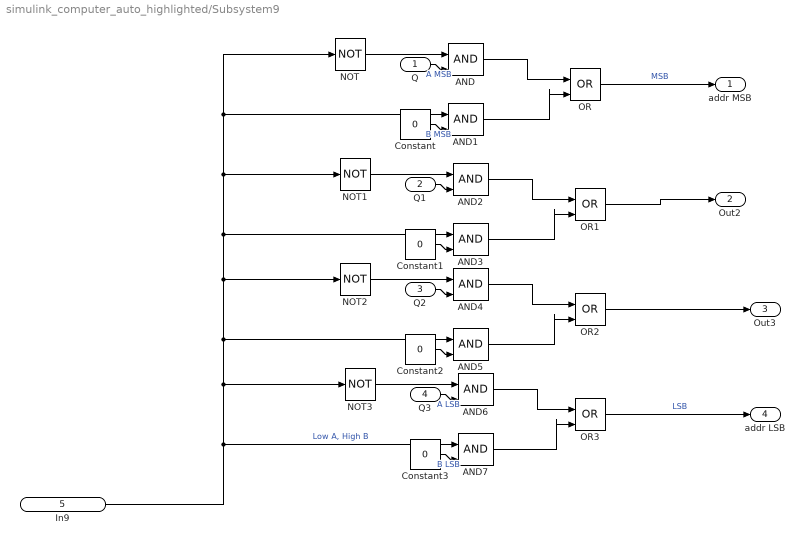
== system simulink_computer_auto_highlighted/Subsystem9 ==
  Q : Inport
  Q1 : Inport  Port=2
  Q2 : Inport  Port=3
  Q3 : Inport  Port=4
  In9 : Inport  Port=5
  AND{,1..7} (8 alike) : Logic  IconShape=distinctive  AllPortsSameDT=off  OutDataTypeStr=boolean
  Constant{,1..3} (4 alike) : Constant  Value=0
  NOT{,1..3} (4 alike) : Logic  Operator=NOT  IconShape=distinctive  AllPortsSameDT=off  OutDataTypeStr=boolean
  OR{,1..3} (4 alike) : Logic  Operator=OR  IconShape=distinctive  AllPortsSameDT=off  OutDataTypeStr=fixdt(1,16)
  addr MSB : Outport  OutDataTypeStr=int16  LockScale=on
  Out2 : Outport  Port=2  OutDataTypeStr=int16  LockScale=on
  Out3 : Outport  Port=3  OutDataTypeStr=int16  LockScale=on
  addr LSB : Outport  Port=4  OutDataTypeStr=int16  LockScale=on
  wires:
  In9/1 -> AND7/1, NOT3/1, AND5/1, NOT2/1, NOT1/1, AND1/1, NOT/1, AND3/1  "Low A, High B"
  AND5/1 -> OR2/2
  NOT/1 -> AND/1
  NOT1/1 -> AND2/1
  AND/1 -> OR/1
  AND2/1 -> OR1/1
  Constant1/1 -> AND3/2
  NOT2/1 -> AND4/1
  AND3/1 -> OR1/2
  AND4/1 -> OR2/1
  OR1/1 -> Out2/1
  Q2/1 -> AND4/2
  AND7/1 -> OR3/2
  AND1/1 -> OR/2
  OR/1 -> addr MSB/1  "MSB"
  AND6/1 -> OR3/1
  Q1/1 -> AND2/2
  OR2/1 -> Out3/1
  NOT3/1 -> AND6/1
  Constant/1 -> AND1/2  "B MSB"
  Constant2/1 -> AND5/2
  Q/1 -> AND/2  "A MSB"
  Constant3/1 -> AND7/2  "B LSB"
  Q3/1 -> AND6/2  "A LSB"
  OR3/1 -> addr LSB/1  "LSB"

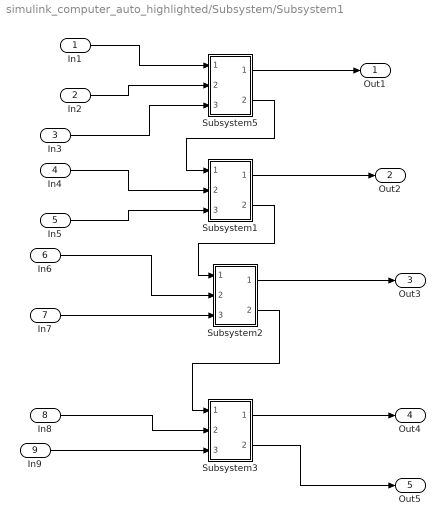
== system simulink_computer_auto_highlighted/Subsystem/Subsystem1 ==
  In1 : Inport
  In2 : Inport  Port=2
  In3 : Inport  Port=3
  In4 : Inport  Port=4
  In5 : Inport  Port=5
  In6 : Inport  Port=6
  In7 : Inport  Port=7
  In8 : Inport  Port=8
  In9 : Inport  Port=9
  Subsystem1 : Subsystem
  Subsystem2 : Subsystem
  Subsystem3 : Subsystem
  Subsystem5 : Subsystem
  Out1 : Outport
  Out2 : Outport  Port=2
  Out3 : Outport  Port=3
  Out4 : Outport  Port=4
  Out5 : Outport  Port=5
  wires:
  Subsystem2/2(Out2) -> Subsystem3/1(In1)
  In8/1 -> Subsystem3/2(In2)
  Subsystem5/2(Out2) -> Subsystem1/1(In1)
  Subsystem2/1(Out1) -> Out3/1
  Subsystem1/2(Out2) -> Subsystem2/1(In1)
  In6/1 -> Subsystem2/2(In2)
  In7/1 -> Subsystem2/3(In3)
  In4/1 -> Subsystem1/2(In2)
  Subsystem3/1(Out1) -> Out4/1
  In9/1 -> Subsystem3/3(In3)
  In2/1 -> Subsystem5/2(In2)
  In3/1 -> Subsystem5/3(In3)
  In1/1 -> Subsystem5/1(In1)
  Subsystem5/1(Out1) -> Out1/1
  Subsystem3/2(Out2) -> Out5/1
  Subsystem1/1(Out1) -> Out2/1
  In5/1 -> Subsystem1/3(In3)

== system simulink_computer_auto_highlighted/Subsystem14/Subsystem4 ==
  In1 : Inport
  In2 : Inport  Port=2
  In3 : Inport  Port=3
  In4 : Inport  Port=4
  AND : Logic  IconShape=distinctive  AllPortsSameDT=off  OutDataTypeStr=boolean
  AND1 : Logic  IconShape=distinctive  AllPortsSameDT=off  OutDataTypeStr=boolean
  OR : Logic  Operator=OR  IconShape=distinctive  AllPortsSameDT=off  OutDataTypeStr=boolean
  Out1 : Outport
  wires:
  AND/1 -> OR/1
  AND1/1 -> OR/2
  OR/1 -> Out1/1
  In3/1 -> AND1/1
  In4/1 -> AND1/2
  In2/1 -> AND/2
  In1/1 -> AND/1

== system simulink_computer_auto_highlighted/Subsystem14/Subsystem5 ==
  In2 : Inport
  In1 : Inport  Port=2
  In3 : Inport  Port=3
  In4 : Inport  Port=4
  AND : Logic  IconShape=distinctive  AllPortsSameDT=off  OutDataTypeStr=boolean
  AND1 : Logic  IconShape=distinctive  AllPortsSameDT=off  OutDataTypeStr=boolean
  OR : Logic  Operator=OR  IconShape=distinctive  AllPortsSameDT=off  OutDataTypeStr=boolean
  Out1 : Outport
  wires:
  AND/1 -> OR/1
  AND1/1 -> OR/2
  OR/1 -> Out1/1
  In3/1 -> AND1/1
  In4/1 -> AND1/2
  In2/1 -> AND/2
  In1/1 -> AND/1

== system simulink_computer_auto_highlighted/Subsystem14/Subsystem6 ==
  In1 : Inport
  In2 : Inport  Port=2
  In3 : Inport  Port=3
  In4 : Inport  Port=4
  AND : Logic  IconShape=distinctive  AllPortsSameDT=off  OutDataTypeStr=boolean
  AND1 : Logic  IconShape=distinctive  AllPortsSameDT=off  OutDataTypeStr=boolean
  OR : Logic  Operator=OR  IconShape=distinctive  AllPortsSameDT=off  OutDataTypeStr=boolean
  Out1 : Outport
  wires:
  AND/1 -> OR/1
  AND1/1 -> OR/2
  OR/1 -> Out1/1
  In3/1 -> AND1/1
  In4/1 -> AND1/2
  In2/1 -> AND/2
  In1/1 -> AND/1

== system simulink_computer_auto_highlighted/Subsystem14/Subsystem7 ==
  In1 : Inport
  In2 : Inport  Port=2
  In3 : Inport  Port=3
  In4 : Inport  Port=4
  AND : Logic  IconShape=distinctive  AllPortsSameDT=off  OutDataTypeStr=boolean
  AND1 : Logic  IconShape=distinctive  AllPortsSameDT=off  OutDataTypeStr=boolean
  OR : Logic  Operator=OR  IconShape=distinctive  AllPortsSameDT=off  OutDataTypeStr=boolean
  Out1 : Outport
  wires:
  AND/1 -> OR/1
  AND1/1 -> OR/2
  OR/1 -> Out1/1
  In3/1 -> AND1/1
  In4/1 -> AND1/2
  In2/1 -> AND/2
  In1/1 -> AND/1

== system simulink_computer_auto_highlighted/Subsystem15/Subsystem10 ==
  load : Inport
  select high : Inport  Port=2
  select low : Inport  Port=3
  AND1 : Logic  IconShape=distinctive  AllPortsSameDT=off  OutDataTypeStr=boolean
  AND2 : Logic  IconShape=distinctive  AllPortsSameDT=off  OutDataTypeStr=boolean
  NOT : Logic  Operator=NOT  IconShape=distinctive  AllPortsSameDT=off  OutDataTypeStr=boolean
  OR : Logic  Operator=OR  IconShape=distinctive  AllPortsSameDT=off  OutDataTypeStr=boolean
  Out1 : Outport
  wires:
  select high/1 -> AND1/2
  OR/1 -> Out1/1  "Q"
  AND1/1 -> OR/1
  NOT/1 -> AND2/1
  AND2/1 -> OR/2
  load/1 -> NOT/1, AND1/1
  select low/1 -> AND2/2

== system simulink_computer_auto_highlighted/Subsystem15/Subsystem11 ==
  load : Inport
  select high : Inport  Port=2
  select low : Inport  Port=3
  AND1 : Logic  IconShape=distinctive  AllPortsSameDT=off  OutDataTypeStr=boolean
  AND2 : Logic  IconShape=distinctive  AllPortsSameDT=off  OutDataTypeStr=boolean
  NOT : Logic  Operator=NOT  IconShape=distinctive  AllPortsSameDT=off  OutDataTypeStr=boolean
  OR : Logic  Operator=OR  IconShape=distinctive  AllPortsSameDT=off  OutDataTypeStr=boolean
  Out1 : Outport
  wires:
  select high/1 -> AND1/2
  OR/1 -> Out1/1  "Q"
  AND1/1 -> OR/1
  NOT/1 -> AND2/1
  AND2/1 -> OR/2
  load/1 -> NOT/1, AND1/1
  select low/1 -> AND2/2

== system simulink_computer_auto_highlighted/Subsystem15/Subsystem12 ==
  load : Inport
  select high : Inport  Port=2
  select low : Inport  Port=3
  AND1 : Logic  IconShape=distinctive  AllPortsSameDT=off  OutDataTypeStr=boolean
  AND2 : Logic  IconShape=distinctive  AllPortsSameDT=off  OutDataTypeStr=boolean
  NOT : Logic  Operator=NOT  IconShape=distinctive  AllPortsSameDT=off  OutDataTypeStr=boolean
  OR : Logic  Operator=OR  IconShape=distinctive  AllPortsSameDT=off  OutDataTypeStr=boolean
  Out1 : Outport
  wires:
  select high/1 -> AND1/2
  OR/1 -> Out1/1  "Q"
  AND1/1 -> OR/1
  NOT/1 -> AND2/1
  AND2/1 -> OR/2
  load/1 -> NOT/1, AND1/1
  select low/1 -> AND2/2

== system simulink_computer_auto_highlighted/Subsystem15/Subsystem13 ==
  load : Inport
  select high : Inport  Port=2
  select low : Inport  Port=3
  AND1 : Logic  IconShape=distinctive  AllPortsSameDT=off  OutDataTypeStr=boolean
  AND2 : Logic  IconShape=distinctive  AllPortsSameDT=off  OutDataTypeStr=boolean
  NOT : Logic  Operator=NOT  IconShape=distinctive  AllPortsSameDT=off  OutDataTypeStr=boolean
  OR : Logic  Operator=OR  IconShape=distinctive  AllPortsSameDT=off  OutDataTypeStr=boolean
  Out1 : Outport
  wires:
  select high/1 -> AND1/2
  OR/1 -> Out1/1  "Q"
  AND1/1 -> OR/1
  NOT/1 -> AND2/1
  AND2/1 -> OR/2
  load/1 -> NOT/1, AND1/1
  select low/1 -> AND2/2

== system simulink_computer_auto_highlighted/Subsystem15/Subsystem2 ==
  load : Inport
  select high : Inport  Port=2
  select low : Inport  Port=3
  AND1 : Logic  IconShape=distinctive  AllPortsSameDT=off  OutDataTypeStr=boolean
  AND2 : Logic  IconShape=distinctive  AllPortsSameDT=off  OutDataTypeStr=boolean
  NOT : Logic  Operator=NOT  IconShape=distinctive  AllPortsSameDT=off  OutDataTypeStr=boolean
  OR : Logic  Operator=OR  IconShape=distinctive  AllPortsSameDT=off  OutDataTypeStr=boolean
  Out1 : Outport
  wires:
  select high/1 -> AND1/2
  OR/1 -> Out1/1  "Q"
  AND1/1 -> OR/1
  NOT/1 -> AND2/1
  AND2/1 -> OR/2
  load/1 -> NOT/1, AND1/1
  select low/1 -> AND2/2

== system simulink_computer_auto_highlighted/Subsystem15/Subsystem3 ==
  load : Inport
  select high : Inport  Port=2
  select low : Inport  Port=3
  AND1 : Logic  IconShape=distinctive  AllPortsSameDT=off  OutDataTypeStr=boolean
  AND2 : Logic  IconShape=distinctive  AllPortsSameDT=off  OutDataTypeStr=boolean
  NOT : Logic  Operator=NOT  IconShape=distinctive  AllPortsSameDT=off  OutDataTypeStr=boolean
  OR : Logic  Operator=OR  IconShape=distinctive  AllPortsSameDT=off  OutDataTypeStr=boolean
  Out1 : Outport
  wires:
  select high/1 -> AND1/2
  OR/1 -> Out1/1  "Q"
  AND1/1 -> OR/1
  NOT/1 -> AND2/1
  AND2/1 -> OR/2
  load/1 -> NOT/1, AND1/1
  select low/1 -> AND2/2

== system simulink_computer_auto_highlighted/Subsystem15/Subsystem4 ==
  load : Inport
  select high : Inport  Port=2
  select low : Inport  Port=3
  AND1 : Logic  IconShape=distinctive  AllPortsSameDT=off  OutDataTypeStr=boolean
  AND2 : Logic  IconShape=distinctive  AllPortsSameDT=off  OutDataTypeStr=boolean
  NOT : Logic  Operator=NOT  IconShape=distinctive  AllPortsSameDT=off  OutDataTypeStr=boolean
  OR : Logic  Operator=OR  IconShape=distinctive  AllPortsSameDT=off  OutDataTypeStr=boolean
  Out1 : Outport
  wires:
  select high/1 -> AND1/2
  OR/1 -> Out1/1  "Q"
  AND1/1 -> OR/1
  NOT/1 -> AND2/1
  AND2/1 -> OR/2
  load/1 -> NOT/1, AND1/1
  select low/1 -> AND2/2

== system simulink_computer_auto_highlighted/Subsystem15/Subsystem5 ==
  load : Inport
  select high : Inport  Port=2
  select low : Inport  Port=3
  AND1 : Logic  IconShape=distinctive  AllPortsSameDT=off  OutDataTypeStr=boolean
  AND2 : Logic  IconShape=distinctive  AllPortsSameDT=off  OutDataTypeStr=boolean
  NOT : Logic  Operator=NOT  IconShape=distinctive  AllPortsSameDT=off  OutDataTypeStr=boolean
  OR : Logic  Operator=OR  IconShape=distinctive  AllPortsSameDT=off  OutDataTypeStr=boolean
  Out1 : Outport
  wires:
  select high/1 -> AND1/2
  OR/1 -> Out1/1  "Q"
  AND1/1 -> OR/1
  NOT/1 -> AND2/1
  AND2/1 -> OR/2
  load/1 -> NOT/1, AND1/1
  select low/1 -> AND2/2

== system simulink_computer_auto_highlighted/Subsystem15/Subsystem6 ==
  load : Inport
  select high : Inport  Port=2
  select low : Inport  Port=3
  AND1 : Logic  IconShape=distinctive  AllPortsSameDT=off  OutDataTypeStr=boolean
  AND2 : Logic  IconShape=distinctive  AllPortsSameDT=off  OutDataTypeStr=boolean
  NOT : Logic  Operator=NOT  IconShape=distinctive  AllPortsSameDT=off  OutDataTypeStr=boolean
  OR : Logic  Operator=OR  IconShape=distinctive  AllPortsSameDT=off  OutDataTypeStr=boolean
  Out1 : Outport
  wires:
  select high/1 -> AND1/2
  OR/1 -> Out1/1  "Q"
  AND1/1 -> OR/1
  NOT/1 -> AND2/1
  AND2/1 -> OR/2
  load/1 -> NOT/1, AND1/1
  select low/1 -> AND2/2

== system simulink_computer_auto_highlighted/Subsystem15/Subsystem7 ==
  load : Inport
  select high : Inport  Port=2
  select low : Inport  Port=3
  AND1 : Logic  IconShape=distinctive  AllPortsSameDT=off  OutDataTypeStr=boolean
  AND2 : Logic  IconShape=distinctive  AllPortsSameDT=off  OutDataTypeStr=boolean
  NOT : Logic  Operator=NOT  IconShape=distinctive  AllPortsSameDT=off  OutDataTypeStr=boolean
  OR : Logic  Operator=OR  IconShape=distinctive  AllPortsSameDT=off  OutDataTypeStr=boolean
  Out1 : Outport
  wires:
  select high/1 -> AND1/2
  OR/1 -> Out1/1  "Q"
  AND1/1 -> OR/1
  NOT/1 -> AND2/1
  AND2/1 -> OR/2
  load/1 -> NOT/1, AND1/1
  select low/1 -> AND2/2

== system simulink_computer_auto_highlighted/Subsystem15/Subsystem8 ==
  load : Inport
  select high : Inport  Port=2
  select low : Inport  Port=3
  AND1 : Logic  IconShape=distinctive  AllPortsSameDT=off  OutDataTypeStr=boolean
  AND2 : Logic  IconShape=distinctive  AllPortsSameDT=off  OutDataTypeStr=boolean
  NOT : Logic  Operator=NOT  IconShape=distinctive  AllPortsSameDT=off  OutDataTypeStr=boolean
  OR : Logic  Operator=OR  IconShape=distinctive  AllPortsSameDT=off  OutDataTypeStr=boolean
  Out1 : Outport
  wires:
  select high/1 -> AND1/2
  OR/1 -> Out1/1  "Q"
  AND1/1 -> OR/1
  NOT/1 -> AND2/1
  AND2/1 -> OR/2
  load/1 -> NOT/1, AND1/1
  select low/1 -> AND2/2

== system simulink_computer_auto_highlighted/Subsystem15/Subsystem9 ==
  load : Inport
  select high : Inport  Port=2
  select low : Inport  Port=3
  AND1 : Logic  IconShape=distinctive  AllPortsSameDT=off  OutDataTypeStr=boolean
  AND2 : Logic  IconShape=distinctive  AllPortsSameDT=off  OutDataTypeStr=boolean
  NOT : Logic  Operator=NOT  IconShape=distinctive  AllPortsSameDT=off  OutDataTypeStr=boolean
  OR : Logic  Operator=OR  IconShape=distinctive  AllPortsSameDT=off  OutDataTypeStr=boolean
  Out1 : Outport
  wires:
  select high/1 -> AND1/2
  OR/1 -> Out1/1  "Q"
  AND1/1 -> OR/1
  NOT/1 -> AND2/1
  AND2/1 -> OR/2
  load/1 -> NOT/1, AND1/1
  select low/1 -> AND2/2

== system simulink_computer_auto_highlighted/Subsystem16/Subsystem4 ==
  In1 : Inport
  In2 : Inport  Port=2
  In3 : Inport  Port=3
  In4 : Inport  Port=4
  AND : Logic  IconShape=distinctive  AllPortsSameDT=off  OutDataTypeStr=boolean
  AND1 : Logic  IconShape=distinctive  AllPortsSameDT=off  OutDataTypeStr=boolean
  OR : Logic  Operator=OR  IconShape=distinctive  AllPortsSameDT=off  OutDataTypeStr=boolean
  Out1 : Outport
  wires:
  AND/1 -> OR/1
  AND1/1 -> OR/2
  OR/1 -> Out1/1
  In3/1 -> AND1/1
  In4/1 -> AND1/2
  In2/1 -> AND/2
  In1/1 -> AND/1

== system simulink_computer_auto_highlighted/Subsystem16/Subsystem5 ==
  In2 : Inport
  In1 : Inport  Port=2
  In3 : Inport  Port=3
  In4 : Inport  Port=4
  AND : Logic  IconShape=distinctive  AllPortsSameDT=off  OutDataTypeStr=boolean
  AND1 : Logic  IconShape=distinctive  AllPortsSameDT=off  OutDataTypeStr=boolean
  OR : Logic  Operator=OR  IconShape=distinctive  AllPortsSameDT=off  OutDataTypeStr=boolean
  Out1 : Outport
  wires:
  AND/1 -> OR/1
  AND1/1 -> OR/2
  OR/1 -> Out1/1
  In3/1 -> AND1/1
  In4/1 -> AND1/2
  In2/1 -> AND/2
  In1/1 -> AND/1

== system simulink_computer_auto_highlighted/Subsystem16/Subsystem6 ==
  In1 : Inport
  In2 : Inport  Port=2
  In3 : Inport  Port=3
  In4 : Inport  Port=4
  AND : Logic  IconShape=distinctive  AllPortsSameDT=off  OutDataTypeStr=boolean
  AND1 : Logic  IconShape=distinctive  AllPortsSameDT=off  OutDataTypeStr=boolean
  OR : Logic  Operator=OR  IconShape=distinctive  AllPortsSameDT=off  OutDataTypeStr=boolean
  Out1 : Outport
  wires:
  AND/1 -> OR/1
  AND1/1 -> OR/2
  OR/1 -> Out1/1
  In3/1 -> AND1/1
  In4/1 -> AND1/2
  In2/1 -> AND/2
  In1/1 -> AND/1

== system simulink_computer_auto_highlighted/Subsystem16/Subsystem7 ==
  In1 : Inport
  In2 : Inport  Port=2
  In3 : Inport  Port=3
  In4 : Inport  Port=4
  AND : Logic  IconShape=distinctive  AllPortsSameDT=off  OutDataTypeStr=boolean
  AND1 : Logic  IconShape=distinctive  AllPortsSameDT=off  OutDataTypeStr=boolean
  OR : Logic  Operator=OR  IconShape=distinctive  AllPortsSameDT=off  OutDataTypeStr=boolean
  Out1 : Outport
  wires:
  AND/1 -> OR/1
  AND1/1 -> OR/2
  OR/1 -> Out1/1
  In3/1 -> AND1/1
  In4/1 -> AND1/2
  In2/1 -> AND/2
  In1/1 -> AND/1

== system simulink_computer_auto_highlighted/Subsystem4/Subsystem4 ==
  In1 : Inport
  In2 : Inport  Port=2
  In3 : Inport  Port=3
  In4 : Inport  Port=4
  AND : Logic  IconShape=distinctive  AllPortsSameDT=off  OutDataTypeStr=boolean
  AND1 : Logic  IconShape=distinctive  AllPortsSameDT=off  OutDataTypeStr=boolean
  OR : Logic  Operator=OR  IconShape=distinctive  AllPortsSameDT=off  OutDataTypeStr=boolean
  Out1 : Outport
  wires:
  AND/1 -> OR/1
  AND1/1 -> OR/2
  OR/1 -> Out1/1
  In3/1 -> AND1/1
  In4/1 -> AND1/2
  In2/1 -> AND/2
  In1/1 -> AND/1

== system simulink_computer_auto_highlighted/Subsystem4/Subsystem5 ==
  In2 : Inport
  In1 : Inport  Port=2
  In3 : Inport  Port=3
  In4 : Inport  Port=4
  AND : Logic  IconShape=distinctive  AllPortsSameDT=off  OutDataTypeStr=boolean
  AND1 : Logic  IconShape=distinctive  AllPortsSameDT=off  OutDataTypeStr=boolean
  OR : Logic  Operator=OR  IconShape=distinctive  AllPortsSameDT=off  OutDataTypeStr=boolean
  Out1 : Outport
  wires:
  AND/1 -> OR/1
  AND1/1 -> OR/2
  OR/1 -> Out1/1
  In3/1 -> AND1/1
  In4/1 -> AND1/2
  In2/1 -> AND/2
  In1/1 -> AND/1

== system simulink_computer_auto_highlighted/Subsystem4/Subsystem6 ==
  In1 : Inport
  In2 : Inport  Port=2
  In3 : Inport  Port=3
  In4 : Inport  Port=4
  AND : Logic  IconShape=distinctive  AllPortsSameDT=off  OutDataTypeStr=boolean
  AND1 : Logic  IconShape=distinctive  AllPortsSameDT=off  OutDataTypeStr=boolean
  OR : Logic  Operator=OR  IconShape=distinctive  AllPortsSameDT=off  OutDataTypeStr=boolean
  Out1 : Outport
  wires:
  AND/1 -> OR/1
  AND1/1 -> OR/2
  OR/1 -> Out1/1
  In3/1 -> AND1/1
  In4/1 -> AND1/2
  In2/1 -> AND/2
  In1/1 -> AND/1

== system simulink_computer_auto_highlighted/Subsystem4/Subsystem7 ==
  In1 : Inport
  In2 : Inport  Port=2
  In3 : Inport  Port=3
  In4 : Inport  Port=4
  AND : Logic  IconShape=distinctive  AllPortsSameDT=off  OutDataTypeStr=boolean
  AND1 : Logic  IconShape=distinctive  AllPortsSameDT=off  OutDataTypeStr=boolean
  OR : Logic  Operator=OR  IconShape=distinctive  AllPortsSameDT=off  OutDataTypeStr=boolean
  Out1 : Outport
  wires:
  AND/1 -> OR/1
  AND1/1 -> OR/2
  OR/1 -> Out1/1
  In3/1 -> AND1/1
  In4/1 -> AND1/2
  In2/1 -> AND/2
  In1/1 -> AND/1

== system simulink_computer_auto_highlighted/Subsystem5/Subsystem4 ==
  In1 : Inport
  In2 : Inport  Port=2
  In3 : Inport  Port=3
  In4 : Inport  Port=4
  AND : Logic  IconShape=distinctive  AllPortsSameDT=off  OutDataTypeStr=boolean
  AND1 : Logic  IconShape=distinctive  AllPortsSameDT=off  OutDataTypeStr=boolean
  OR : Logic  Operator=OR  IconShape=distinctive  AllPortsSameDT=off  OutDataTypeStr=boolean
  Out1 : Outport
  wires:
  AND/1 -> OR/1
  AND1/1 -> OR/2
  OR/1 -> Out1/1
  In3/1 -> AND1/1
  In4/1 -> AND1/2
  In2/1 -> AND/2
  In1/1 -> AND/1

== system simulink_computer_auto_highlighted/Subsystem5/Subsystem5 ==
  In2 : Inport
  In1 : Inport  Port=2
  In3 : Inport  Port=3
  In4 : Inport  Port=4
  AND : Logic  IconShape=distinctive  AllPortsSameDT=off  OutDataTypeStr=boolean
  AND1 : Logic  IconShape=distinctive  AllPortsSameDT=off  OutDataTypeStr=boolean
  OR : Logic  Operator=OR  IconShape=distinctive  AllPortsSameDT=off  OutDataTypeStr=boolean
  Out1 : Outport
  wires:
  AND/1 -> OR/1
  AND1/1 -> OR/2
  OR/1 -> Out1/1
  In3/1 -> AND1/1
  In4/1 -> AND1/2
  In2/1 -> AND/2
  In1/1 -> AND/1

== system simulink_computer_auto_highlighted/Subsystem5/Subsystem6 ==
  In1 : Inport
  In2 : Inport  Port=2
  In3 : Inport  Port=3
  In4 : Inport  Port=4
  AND : Logic  IconShape=distinctive  AllPortsSameDT=off  OutDataTypeStr=boolean
  AND1 : Logic  IconShape=distinctive  AllPortsSameDT=off  OutDataTypeStr=boolean
  OR : Logic  Operator=OR  IconShape=distinctive  AllPortsSameDT=off  OutDataTypeStr=boolean
  Out1 : Outport
  wires:
  AND/1 -> OR/1
  AND1/1 -> OR/2
  OR/1 -> Out1/1
  In3/1 -> AND1/1
  In4/1 -> AND1/2
  In2/1 -> AND/2
  In1/1 -> AND/1

== system simulink_computer_auto_highlighted/Subsystem5/Subsystem7 ==
  In1 : Inport
  In2 : Inport  Port=2
  In3 : Inport  Port=3
  In4 : Inport  Port=4
  AND : Logic  IconShape=distinctive  AllPortsSameDT=off  OutDataTypeStr=boolean
  AND1 : Logic  IconShape=distinctive  AllPortsSameDT=off  OutDataTypeStr=boolean
  OR : Logic  Operator=OR  IconShape=distinctive  AllPortsSameDT=off  OutDataTypeStr=boolean
  Out1 : Outport
  wires:
  AND/1 -> OR/1
  AND1/1 -> OR/2
  OR/1 -> Out1/1
  In3/1 -> AND1/1
  In4/1 -> AND1/2
  In2/1 -> AND/2
  In1/1 -> AND/1

== system simulink_computer_auto_highlighted/Subsystem8/Subsystem1 ==
  In1 : Inport
  Demux : Demux
  MATLAB Function : MATLAB Function  TreatAsAtomicUnit=on
  y : Outport
  wires:
  Demux/3 -> MATLAB Function/3(b1)
  Demux/1 -> MATLAB Function/1(b3)
  Demux/2 -> MATLAB Function/2(b2)
  Demux/4 -> MATLAB Function/4(b0)
  MATLAB Function/1(y) -> y/1
  In1/1 -> Demux/1

== system simulink_computer_auto_highlighted/Subsystem/Subsystem1/Subsystem1 ==
  In1 : Inport
  In2 : Inport  Port=2
  In3 : Inport  Port=3
  AND : Logic  IconShape=distinctive  AllPortsSameDT=off  OutDataTypeStr=boolean
  AND1 : Logic  IconShape=distinctive  AllPortsSameDT=off  OutDataTypeStr=boolean
  OR : Logic  Operator=OR  IconShape=distinctive  AllPortsSameDT=off  OutDataTypeStr=boolean
  XOR : Logic  Operator=XOR  IconShape=distinctive  AllPortsSameDT=off  OutDataTypeStr=boolean
  XOR1 : Logic  Operator=XOR  IconShape=distinctive  AllPortsSameDT=off  OutDataTypeStr=boolean
  Out1 : Outport
  Out2 : Outport  Port=2
  wires:
  AND1/1 -> OR/1
  AND/1 -> OR/2
  In3/1 -> AND/2, XOR/2
  In2/1 -> AND/1, XOR/1
  In1/1 -> XOR1/2, AND1/2
  XOR/1 -> AND1/1, XOR1/1
  XOR1/1 -> Out1/1
  OR/1 -> Out2/1

== system simulink_computer_auto_highlighted/Subsystem/Subsystem1/Subsystem2 ==
  In1 : Inport
  In2 : Inport  Port=2
  In3 : Inport  Port=3
  AND : Logic  IconShape=distinctive  AllPortsSameDT=off  OutDataTypeStr=boolean
  AND1 : Logic  IconShape=distinctive  AllPortsSameDT=off  OutDataTypeStr=boolean
  OR : Logic  Operator=OR  IconShape=distinctive  AllPortsSameDT=off  OutDataTypeStr=boolean
  XOR : Logic  Operator=XOR  IconShape=distinctive  AllPortsSameDT=off  OutDataTypeStr=boolean
  XOR1 : Logic  Operator=XOR  IconShape=distinctive  AllPortsSameDT=off  OutDataTypeStr=boolean
  Out1 : Outport
  Out2 : Outport  Port=2
  wires:
  AND1/1 -> OR/1
  AND/1 -> OR/2
  In3/1 -> AND/2, XOR/2
  In2/1 -> AND/1, XOR/1
  In1/1 -> XOR1/2, AND1/2
  XOR/1 -> AND1/1, XOR1/1
  XOR1/1 -> Out1/1
  OR/1 -> Out2/1
